simulink model "Get_Horizontal_Measures"  (R2014a)
settings: configuration reference "AR_Drone_ConfigSet" (kept outside this file)
undefined symbols (not defined in the file or in its folder): Accelerometer_360deg_calibration, Magnetometer_calibration, Navigation, Navigation_KF_Lib
libraries: simulink x7, AR_Drone_2_Library x1, vrlib x1
settings Model: SimulationMode=external  ExtModeTrigDuration=48000  Creator=nraman  LastModifiedBy=Raphaël

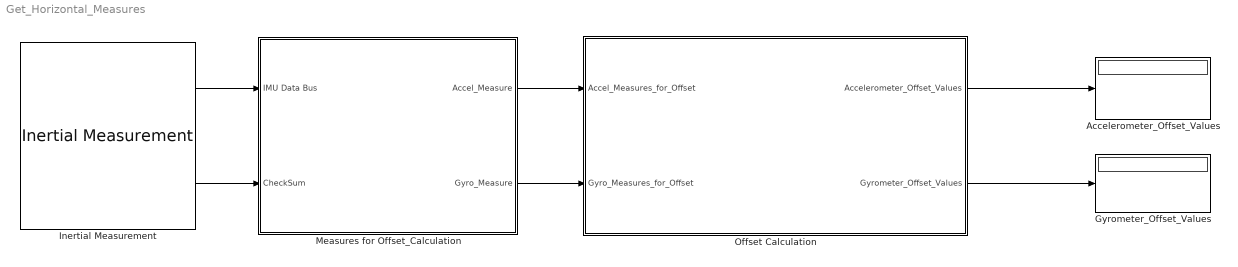
== system Get_Horizontal_Measures ==
  Accelerometer_Offset_Values : Display
      settings: Decimation=3
  Gyrometer_Offset_Values : Display
      settings: Decimation=3
  Inertial Measurement : AR_Drone_2_Library/Inertial Measurement  Ts=1/400
  Measures for Offset_Calculation : Subsystem  AncestorBlock=Navigation_KF_Lib/Navigation
      mask DialogControl DescTextVar Prompt: Kalman Filter Navigation Implementation
  Offset Calculation : Stateflow chart  RequirementInfo="{}  %GIDa_de274cbe_aff3_43d2_a93a_eae542baa43c"  TreatAsAtomicUnit=on
  wires:
  Inertial Measurement/1 -> Measures for Offset_Calculation/1(IMU Data Bus)
  Inertial Measurement/2 -> Measures for Offset_Calculation/2(CheckSum)
  Measures for Offset_Calculation/1(Accel_Measure) -> Offset Calculation/1(Accel_Measures_for_Offset)
  Measures for Offset_Calculation/2(Gyro_Measure) -> Offset Calculation/2(Gyro_Measures_for_Offset)
  Offset Calculation/2(Gyrometer_Offset_Values) -> Gyrometer_Offset_Values/1
  Offset Calculation/1(Accelerometer_Offset_Values) -> Accelerometer_Offset_Values/1

== system Get_Horizontal_Measures/Measures for Offset_Calculation ==
  IMU Data Bus : Inport  OutDataTypeStr=Bus: IMU_Packets
  CheckSum : Inport  Port=2
  Bus Creator1 : BusCreator  Inputs=5
  CheckSum Pre-Processing : Subsystem  TreatAsAtomicUnit=on
      settings: RTWSystemCode=Inline
  Data Conversion and Measurement Calculation : Subsystem
  Accel_Measure : Outport
  Gyro_Measure : Outport  Port=2
  wires:
  Bus Creator1/1 -> Data Conversion and Measurement Calculation/1(MeasurementDataBus)
  CheckSum Pre-Processing/5(GyroTemp_Measure) -> Bus Creator1/5  "GyroTemp_Measure"
  CheckSum Pre-Processing/4(Accelerometer_Measure) -> Bus Creator1/4  "Accelerometer_Measure"
  CheckSum Pre-Processing/3(BodyRates_Measure) -> Bus Creator1/3  "BodyRates_Measure"
  CheckSum Pre-Processing/2(Magnetometer_Measure) -> Bus Creator1/2  "Magnetometer_Measure"
  CheckSum Pre-Processing/1(UltraSoundHeight_Measure) -> Bus Creator1/1  "Ultrasound_Measure"
  CheckSum/1 -> CheckSum Pre-Processing/2(CheckSumFlag)
  IMU Data Bus/1 -> CheckSum Pre-Processing/1(IMU Packets)
  Data Conversion and Measurement Calculation/1(Accel_Measure) -> Accel_Measure/1
  Data Conversion and Measurement Calculation/2(Gyro_Measure) -> Gyro_Measure/1

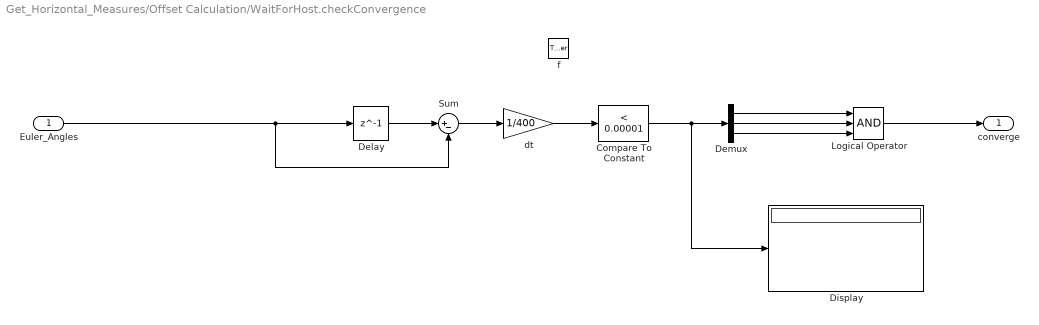
== system Get_Horizontal_Measures/Offset Calculation/WaitForHost.checkConvergence ==
  Euler_Angles : Inport  OutDataTypeStr=double  PortDimensions=3
  f : TriggerPort  TriggerType=function-call
      settings: CopyFcn=Stateflow.SLINSF.SimulinkMan.removeBlockPreDeleteFcn  PreDeleteFcn=Stateflow.SLINSF.SimulinkMan.unsafePredeleteFcn
  Compare To Constant : simulink/Logic and Bit Operations/Compare To Constant  relop=<  const=0.00001  OutDataTypeStr=boolean
  Delay : Delay  DelayLength=1  InitialCondition=inf
  Demux : Demux  Outputs=3
  Display : Display
  Logical Operator : Logic  Inputs=3  AllPortsSameDT=off  OutDataTypeStr=boolean
  Sum : Sum  Inputs=|+-
  dt : Gain  Gain=1/400
  converge : Outport
  wires:
  Euler_Angles/1 -> Sum/2, Delay/1
  Delay/1 -> Sum/1
  Sum/1 -> dt/1
  dt/1 -> Compare To Constant/1
  Compare To Constant/1 -> Display/1, Demux/1
  Logical Operator/1 -> converge/1
  Demux/1 -> Logical Operator/1
  Demux/2 -> Logical Operator/2
  Demux/3 -> Logical Operator/3

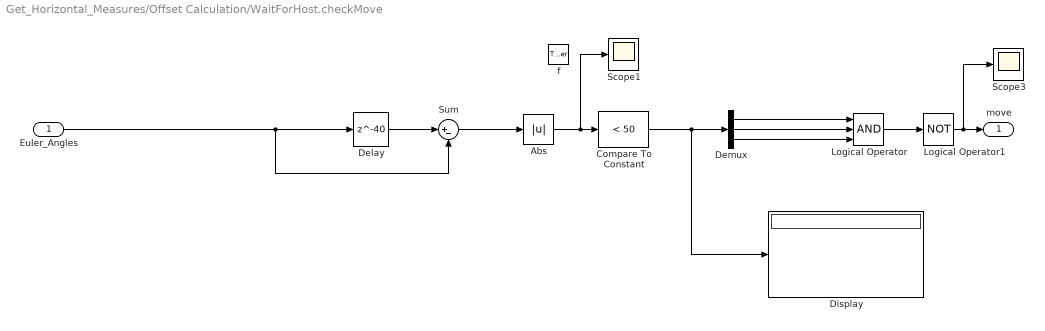
== system Get_Horizontal_Measures/Offset Calculation/WaitForHost.checkMove ==
  Euler_Angles : Inport  OutDataTypeStr=double  PortDimensions=3
  f : TriggerPort  TriggerType=function-call
      settings: CopyFcn=Stateflow.SLINSF.SimulinkMan.removeBlockPreDeleteFcn  PreDeleteFcn=Stateflow.SLINSF.SimulinkMan.unsafePredeleteFcn
  Abs : Abs
  Compare To Constant : simulink/Logic and Bit Operations/Compare To Constant  relop=<  const=50  OutDataTypeStr=boolean
  Delay : Delay  DelayLength=40  InitialCondition=inf
  Demux : Demux  Outputs=3
  Display : Display
  Logical Operator : Logic  Inputs=3  AllPortsSameDT=off  OutDataTypeStr=boolean
  Logical Operator1 : Logic  Operator=NOT  AllPortsSameDT=off  OutDataTypeStr=boolean
  Scope1 : Scope
      settings: SaveName=Difference
  Scope3 : Scope
      settings: SaveName=Move
  Sum : Sum  Inputs=|+-
  move : Outport
  wires:
  Euler_Angles/1 -> Sum/2, Delay/1
  Delay/1 -> Sum/1
  Sum/1 -> Abs/1
  Compare To Constant/1 -> Display/1, Demux/1
  Logical Operator/1 -> Logical Operator1/1
  Demux/1 -> Logical Operator/1
  Demux/2 -> Logical Operator/2
  Demux/3 -> Logical Operator/3
  Logical Operator1/1 -> Scope3/1, move/1
  Abs/1 -> Scope1/1, Compare To Constant/1

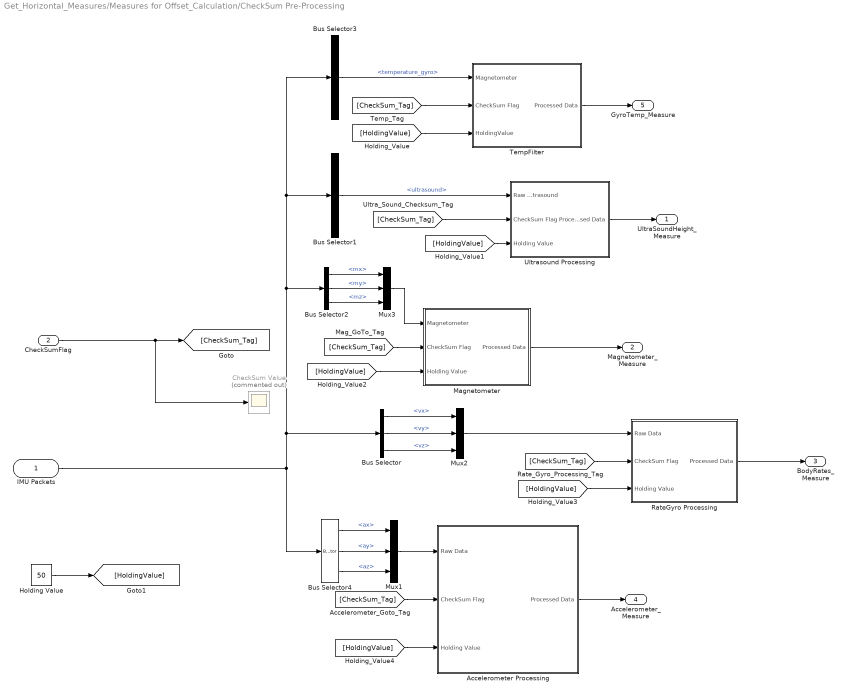
== system Get_Horizontal_Measures/Measures for Offset_Calculation/CheckSum Pre-Processing ==
  IMU Packets : Inport
  CheckSumFlag : Inport  Port=2
  Accelerometer Processing : Subsystem
  Bus Selector : BusSelector  OutputSignals=vx,vy,vz
  Bus Selector1 : BusSelector  OutputSignals=ultrasound
  Bus Selector2 : BusSelector  OutputSignals=mx,my,mz
  Bus Selector3 : BusSelector  OutputSignals=temperature_gyro
  Bus Selector4 : BusSelector  OutputSignals=ax,ay,az
  CheckSum Value : Scope  Commented=on
      settings: YMin=0  YMax=2500  SaveName=CheckSum
  Holding Value : Constant  Value=50
  Magnetometer : Subsystem
  Mux1 : Mux  Inputs=3
  Mux2 : Mux  Inputs=3
  Mux3 : Mux  Inputs=3
  RateGyro Processing : Subsystem
  TempFilter : Subsystem
  Ultrasound Processing : Subsystem
  UltraSoundHeight_Measure : Outport
  Magnetometer_Measure : Outport  Port=2
  BodyRates_Measure : Outport  Port=3
  Accelerometer_Measure : Outport  Port=4
  GyroTemp_Measure : Outport  Port=5
  wires:
  Mux3/1 -> Magnetometer/1(Magnetometer)
  Holding Value/1 -> [HoldingValue]
  [HoldingValue] -> Accelerometer Processing/3(Holding Value)
  [HoldingValue] -> RateGyro Processing/3(Holding Value)
  [HoldingValue] -> Magnetometer/3(Holding Value)
  [HoldingValue] -> Ultrasound Processing/3(Holding Value)
  [HoldingValue] -> TempFilter/3(HoldingValue)
  [CheckSum_Tag] -> TempFilter/2(CheckSum Flag)
  TempFilter/1(Processed Data) -> GyroTemp_Measure/1
  Bus Selector3/1 -> TempFilter/1(Magnetometer)  "<temperature_gyro>"
  Bus Selector/3 -> Mux2/3  "<vz>"
  Bus Selector/2 -> Mux2/2  "<vy>"
  Bus Selector/1 -> Mux2/1  "<vx>"
  Ultrasound Processing/1(Processed Data) -> UltraSoundHeight_Measure/1
  [CheckSum_Tag] -> Accelerometer Processing/2(CheckSum Flag)
  Magnetometer/1(Processed Data) -> Magnetometer_Measure/1
  [CheckSum_Tag] -> Magnetometer/2(CheckSum Flag)
  Bus Selector2/3 -> Mux3/3  "<mz>"
  Bus Selector2/2 -> Mux3/2  "<my>"
  Bus Selector2/1 -> Mux3/1  "<mx>"
  RateGyro Processing/1(Processed Data) -> BodyRates_Measure/1
  [CheckSum_Tag] -> RateGyro Processing/2(CheckSum Flag)
  Mux2/1 -> RateGyro Processing/1(Raw Data)
  Accelerometer Processing/1(Processed Data) -> Accelerometer_Measure/1
  [CheckSum_Tag] -> Ultrasound Processing/2(CheckSum Flag)
  Mux1/1 -> Accelerometer Processing/1(Raw Data)
  Bus Selector4/3 -> Mux1/3  "<az>"
  Bus Selector4/2 -> Mux1/2  "<ay>"
  Bus Selector4/1 -> Mux1/1  "<ax>"
  IMU Packets/1 -> Bus Selector4/1, Bus Selector2/1, Bus Selector1/1, Bus Selector3/1, Bus Selector/1
  CheckSumFlag/1 -> CheckSum Value/1, [CheckSum_Tag]
  Bus Selector1/1 -> Ultrasound Processing/1(Raw Ultrasound)  "<ultrasound>"

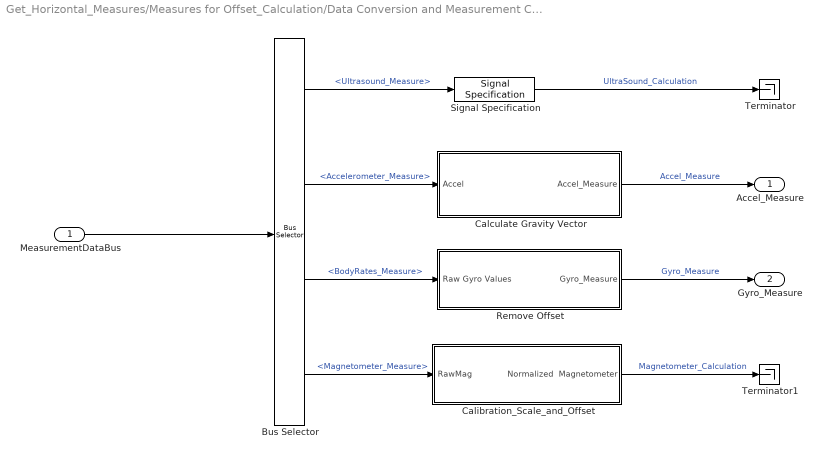
== system Get_Horizontal_Measures/Measures for Offset_Calculation/Data Conversion and Measurement Calculation ==
  MeasurementDataBus : Inport
  Bus Selector : BusSelector  OutputSignals=Ultrasound_Measure,Accelerometer_Measure,BodyRates_Measure,Magnetometer_Measure
  Calculate Gravity Vector : Subsystem
  Calibration_Scale_and_Offset : Subsystem
  Remove Offset : Subsystem
  Signal Specification : SignalSpecification
  Terminator : Terminator
  Terminator1 : Terminator
  Accel_Measure : Outport
  Gyro_Measure : Outport  Port=2
  wires:
  MeasurementDataBus/1 -> Bus Selector/1
  Bus Selector/4 -> Calibration_Scale_and_Offset/1(RawMag)  "<Magnetometer_Measure>"
  Bus Selector/3 -> Remove Offset/1(Raw Gyro Values)  "<BodyRates_Measure>"
  Bus Selector/1 -> Signal Specification/1  "<Ultrasound_Measure>"
  Calibration_Scale_and_Offset/1(Normalized  Magnetometer) -> Terminator1/1  "Magnetometer_Calculation"
  Remove Offset/1(Gyro_Measure) -> Gyro_Measure/1  "Gyro_Measure"
  Signal Specification/1 -> Terminator/1  "UltraSound_Calculation"
  Calculate Gravity Vector/1(Accel_Measure) -> Accel_Measure/1  "Accel_Measure"
  Bus Selector/2 -> Calculate Gravity Vector/1(Accel)  "<Accelerometer_Measure>"

== system Get_Horizontal_Measures/Measures for Offset_Calculation/CheckSum Pre-Processing/Accelerometer Processing ==
  Raw Data : Inport
  CheckSum Flag : Inport  Port=2
  Holding Value : Inport  Port=3
  Calculate Accel Data : Subsystem  Commented=through
  CheckSum Correction : Subsystem
  Processed Data : Outport
  wires:
  Holding Value/1 -> CheckSum Correction/3(Holding Value)
  Calculate Accel Data/1(Processed Accel Data) -> CheckSum Correction/1(CalculatedData)
  CheckSum Correction/1(Pre-Processed Height) -> Processed Data/1
  Raw Data/1 -> Calculate Accel Data/1(Raw Accel Data)
  CheckSum Flag/1 -> CheckSum Correction/2(CheckSumFlag)

== system Get_Horizontal_Measures/Measures for Offset_Calculation/CheckSum Pre-Processing/Magnetometer ==
  Magnetometer : Inport
  CheckSum Flag : Inport  Port=2
  Holding Value : Inport  Port=3
  CheckSum Correction : Subsystem
  Process Raw Mag Data : Subsystem  Commented=through
  Processed Data : Outport
  wires:
  Holding Value/1 -> CheckSum Correction/3(Holding Value)
  Process Raw Mag Data/1(ProcessedData) -> CheckSum Correction/1(CalculatedData)
  Magnetometer/1 -> Process Raw Mag Data/1(Magnetometer)
  CheckSum Correction/1(Pre-Processed Data) -> Processed Data/1
  CheckSum Flag/1 -> CheckSum Correction/2(CheckSumFlag)

== system Get_Horizontal_Measures/Measures for Offset_Calculation/CheckSum Pre-Processing/RateGyro Processing ==
  Raw Data : Inport
  CheckSum Flag : Inport  Port=2
  Holding Value : Inport  Port=3
  CheckSum Correction : Subsystem
  Process Data : Subsystem  Commented=through
  Processed Data : Outport
  wires:
  Holding Value/1 -> CheckSum Correction/3(Holding Value)
  Process Data/1(Processed Data) -> CheckSum Correction/1(CalculatedData)
  Raw Data/1 -> Process Data/1(Raw Data)
  CheckSum Correction/1(Pre-Processed Height) -> Processed Data/1
  CheckSum Flag/1 -> CheckSum Correction/2(CheckSumFlag)

== system Get_Horizontal_Measures/Measures for Offset_Calculation/CheckSum Pre-Processing/TempFilter ==
  Magnetometer : Inport
  CheckSum Flag : Inport  Port=2
  HoldingValue : Inport  Port=3
  CheckSum Correction : Subsystem
  Process Raw Mag Data : Subsystem  Commented=through
  Processed Data : Outport
  wires:
  HoldingValue/1 -> CheckSum Correction/3(Holding Value)
  Process Raw Mag Data/1(ProcessedData) -> CheckSum Correction/1(CalculatedData)
  Magnetometer/1 -> Process Raw Mag Data/1(Magnetometer)
  CheckSum Correction/1(Pre-Processed Data) -> Processed Data/1
  CheckSum Flag/1 -> CheckSum Correction/2(CheckSumFlag)

== system Get_Horizontal_Measures/Measures for Offset_Calculation/CheckSum Pre-Processing/Ultrasound Processing ==
  note: '192.168.1.1' 1 17725
  Raw Ultrasound : Inport
  CheckSum Flag : Inport  Port=2
  Holding Value : Inport  Port=3
  CheckSum Correction : Subsystem
  Data Type Conversion1 : DataTypeConversion
  Delay1 : Delay  DelayLength=1  InitialCondition=0
  Height Calculation : MATLAB Function  TreatAsAtomicUnit=on
  Saturation1 : Saturate  UpperLimit=100e3  LowerLimit=0
  Processed Data : Outport
  wires:
  Holding Value/1 -> CheckSum Correction/3(Holding Value)
  Saturation1/1 -> Processed Data/1
  CheckSum Correction/1(Pre-Processed Height) -> Saturation1/1
  CheckSum Flag/1 -> CheckSum Correction/2(CheckSumFlag)
  Height Calculation/1(y) -> CheckSum Correction/1(CalculatedData)
  Raw Ultrasound/1 -> Data Type Conversion1/1
  Height Calculation/2(prev_good_height) -> Delay1/1
  Data Type Conversion1/1 -> Height Calculation/1(u)
  Delay1/1 -> Height Calculation/2(z_1)

== system Get_Horizontal_Measures/Measures for Offset_Calculation/Data Conversion and Measurement Calculation/Calculate Gravity Vector ==
  Accel : Inport
  Accelerometer Neutral Gain and Offset : Subsystem
  Calibration_GainOffset : Subsystem
  Compare Calibration : Scope  NumInputPorts=2
      settings: TimeRange=6.848856838354834  YMin=-1.05~-1.05  YMax=0.05~0.1  SaveName=AccelProcessed_Record1
  Compare Offset : Scope  NumInputPorts=2
      settings: TimeRange=6.848856838354834  YMin=-0.05~-1  YMax=1.05~0.05  SaveName=AccelProcessed_Record
  InitialCondition_Offset : Subsystem
  Accel_Measure : Outport
  wires:
  Accelerometer Neutral Gain and Offset/1(Processed Accel Data) -> Compare Calibration/2, Calibration_GainOffset/1(Pre)
  Calibration_GainOffset/1(Post) -> Compare Offset/2, Compare Calibration/1, InitialCondition_Offset/1(Pre)
  Accel/1 -> Accelerometer Neutral Gain and Offset/1(Raw Accel Data)
  InitialCondition_Offset/1(Post) -> Accel_Measure/1, Compare Offset/1

== system Get_Horizontal_Measures/Measures for Offset_Calculation/Data Conversion and Measurement Calculation/Calibration_Scale_and_Offset ==
  RawMag : Inport
  Normalize Vector : vrlib/Utilities/Normalize Vector  maxzero=0
  Process Raw Mag Data : Subsystem  Variant=on  OverrideUsingVariant=TempVariantA
  Normalized  Magnetometer : Outport
  wires:
  Process Raw Mag Data/1(MagVector) -> Normalize Vector/1
  RawMag/1 -> Process Raw Mag Data/1(Magnetometer)
  Normalize Vector/1 -> Normalized  Magnetometer/1

== system Get_Horizontal_Measures/Measures for Offset_Calculation/Data Conversion and Measurement Calculation/Remove Offset ==
  Raw Gyro Values : Inport
  Gyro_Measure : Outport
  tag scope: Gyro_data_for_offset=global
  wires:
  Raw Gyro Values/1 -> Gyro_Measure/1, [Gyro_data_for_offset]

== system Get_Horizontal_Measures/Measures for Offset_Calculation/CheckSum Pre-Processing/Accelerometer Processing/Calculate Accel Data ==
  Raw Accel Data : Inport
  Bias : Constant  Value=[0 4096 4096]
  Gain : Gain  Gain=[0.001953125, 0.001953125, 0.001953125]
  Neutral Bias : Constant  Value=[2048 2048 2048]
  Sum : Sum  Inputs=|-+
  Sum1 : Sum  Inputs=|+-
  Processed Accel Data : Outport
  wires:
  Bias/1 -> Sum/2
  Neutral Bias/1 -> Sum1/2
  Sum/1 -> Sum1/1
  Gain/1 -> Processed Accel Data/1
  Sum1/1 -> Gain/1
  Raw Accel Data/1 -> Sum/1

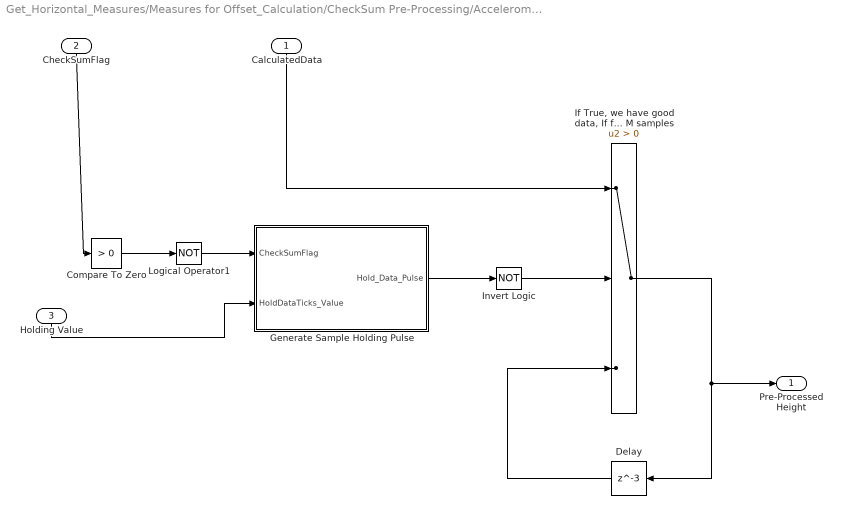
== system Get_Horizontal_Measures/Measures for Offset_Calculation/CheckSum Pre-Processing/Accelerometer Processing/CheckSum Correction ==
  CalculatedData : Inport
  CheckSumFlag : Inport  Port=2
  Holding Value : Inport  Port=3
  Compare To Zero : simulink/Logic and Bit Operations/Compare To Zero  relop=>  OutDataTypeStr=boolean
  Delay : Delay  DelayLength=3  InitialCondition=0
  Generate Sample Holding Pulse : Subsystem
  "If True, we have good data, If false, we have bad data, With bad data, use previous good data from N samples ago and hold it on that value for M samples" : Switch  Criteria=u2 > Threshold
  Invert Logic : Logic  Operator=NOT  AllPortsSameDT=off  OutDataTypeStr=boolean
  Logical Operator1 : Logic  Operator=NOT  AllPortsSameDT=off  OutDataTypeStr=boolean
  Pre-Processed Height : Outport
  wires:
  Holding Value/1 -> Generate Sample Holding Pulse/2(HoldDataTicks_Value)
  Invert Logic/1 -> "If True, we have good data, If false, we have bad data, With bad data, use previous good data from N samples ago and hold it on that value for M samples"/2
  Logical Operator1/1 -> Generate Sample Holding Pulse/1(CheckSumFlag)
  Generate Sample Holding Pulse/1(Hold_Data_Pulse) -> Invert Logic/1
  Compare To Zero/1 -> Logical Operator1/1
  Delay/1 -> "If True, we have good data, If false, we have bad data, With bad data, use previous good data from N samples ago and hold it on that value for M samples"/3
  "If True, we have good data, If false, we have bad data, With bad data, use previous good data from N samples ago and hold it on that value for M samples"/1 -> Delay/1, Pre-Processed Height/1
  CalculatedData/1 -> "If True, we have good data, If false, we have bad data, With bad data, use previous good data from N samples ago and hold it on that value for M samples"/1
  CheckSumFlag/1 -> Compare To Zero/1

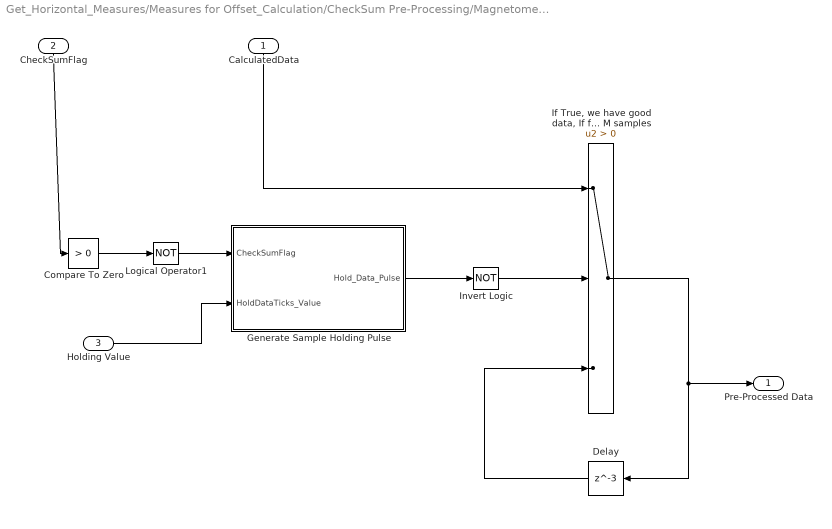
== system Get_Horizontal_Measures/Measures for Offset_Calculation/CheckSum Pre-Processing/Magnetometer/CheckSum Correction ==
  CalculatedData : Inport
  CheckSumFlag : Inport  Port=2
  Holding Value : Inport  Port=3
  Compare To Zero : simulink/Logic and Bit Operations/Compare To Zero  relop=>  OutDataTypeStr=boolean
  Delay : Delay  DelayLength=3  InitialCondition=0
  Generate Sample Holding Pulse : Subsystem
  "If True, we have good data, If false, we have bad data, With bad data, use previous good data from N samples ago and hold it on that value for M samples" : Switch  Criteria=u2 > Threshold
  Invert Logic : Logic  Operator=NOT  AllPortsSameDT=off  OutDataTypeStr=boolean
  Logical Operator1 : Logic  Operator=NOT  AllPortsSameDT=off  OutDataTypeStr=boolean
  Pre-Processed Data : Outport
  wires:
  Holding Value/1 -> Generate Sample Holding Pulse/2(HoldDataTicks_Value)
  Invert Logic/1 -> "If True, we have good data, If false, we have bad data, With bad data, use previous good data from N samples ago and hold it on that value for M samples"/2
  Logical Operator1/1 -> Generate Sample Holding Pulse/1(CheckSumFlag)
  Generate Sample Holding Pulse/1(Hold_Data_Pulse) -> Invert Logic/1
  Compare To Zero/1 -> Logical Operator1/1
  Delay/1 -> "If True, we have good data, If false, we have bad data, With bad data, use previous good data from N samples ago and hold it on that value for M samples"/3
  "If True, we have good data, If false, we have bad data, With bad data, use previous good data from N samples ago and hold it on that value for M samples"/1 -> Delay/1, Pre-Processed Data/1
  CalculatedData/1 -> "If True, we have good data, If false, we have bad data, With bad data, use previous good data from N samples ago and hold it on that value for M samples"/1
  CheckSumFlag/1 -> Compare To Zero/1

== system Get_Horizontal_Measures/Measures for Offset_Calculation/CheckSum Pre-Processing/Magnetometer/Process Raw Mag Data ==
  note: magnetometer[ 0 ] = - ( float ) navdata.mx ;
      | magnetometer[ 1 ] = ( float ) navdata.my ;
      | magnetometer[ 2 ] = - ( float ) navdata.mz ;
      | const float Sensitivity[ 3 ] = { 0.0071492608 , 0.0070882491 , 0.0074057781 } ;
      | const float Neutral[ 3 ] = { 118.0 , - 65.0 , 110.0 } ;
  Magnetometer : Inport
  Bias : Constant  Value=[ 118.0, -65.0, 110.0 ]
  Sum : Sum  Inputs=|+-
  postGain : Gain  Gain=[0.0071492608, 0.0070882491, 0.0074057781]
  preGain : Gain  Gain=[-1 1 -1]
  ProcessedData : Outport
  wires:
  Bias/1 -> Sum/2
  preGain/1 -> Sum/1
  Sum/1 -> postGain/1
  Magnetometer/1 -> preGain/1
  postGain/1 -> ProcessedData/1

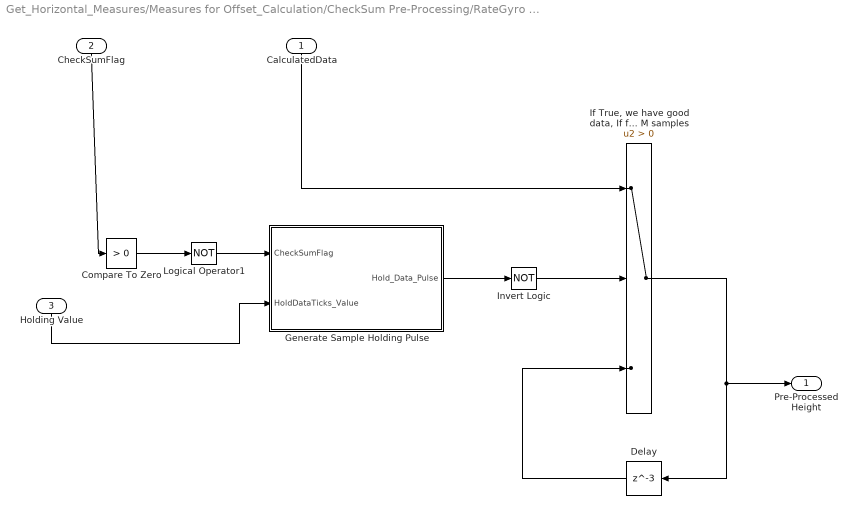
== system Get_Horizontal_Measures/Measures for Offset_Calculation/CheckSum Pre-Processing/RateGyro Processing/CheckSum Correction ==
  CalculatedData : Inport
  CheckSumFlag : Inport  Port=2
  Holding Value : Inport  Port=3
  Compare To Zero : simulink/Logic and Bit Operations/Compare To Zero  relop=>  OutDataTypeStr=boolean
  Delay : Delay  DelayLength=3  InitialCondition=0
  Generate Sample Holding Pulse : Subsystem
  "If True, we have good data, If false, we have bad data, With bad data, use previous good data from N samples ago and hold it on that value for M samples" : Switch  Criteria=u2 > Threshold
  Invert Logic : Logic  Operator=NOT  AllPortsSameDT=off  OutDataTypeStr=boolean
  Logical Operator1 : Logic  Operator=NOT  AllPortsSameDT=off  OutDataTypeStr=boolean
  Pre-Processed Height : Outport
  wires:
  Holding Value/1 -> Generate Sample Holding Pulse/2(HoldDataTicks_Value)
  Invert Logic/1 -> "If True, we have good data, If false, we have bad data, With bad data, use previous good data from N samples ago and hold it on that value for M samples"/2
  Logical Operator1/1 -> Generate Sample Holding Pulse/1(CheckSumFlag)
  Generate Sample Holding Pulse/1(Hold_Data_Pulse) -> Invert Logic/1
  Compare To Zero/1 -> Logical Operator1/1
  Delay/1 -> "If True, we have good data, If false, we have bad data, With bad data, use previous good data from N samples ago and hold it on that value for M samples"/3
  "If True, we have good data, If false, we have bad data, With bad data, use previous good data from N samples ago and hold it on that value for M samples"/1 -> Delay/1, Pre-Processed Height/1
  CalculatedData/1 -> "If True, we have good data, If false, we have bad data, With bad data, use previous good data from N samples ago and hold it on that value for M samples"/1
  CheckSumFlag/1 -> Compare To Zero/1

== system Get_Horizontal_Measures/Measures for Offset_Calculation/CheckSum Pre-Processing/RateGyro Processing/Process Data ==
  note: const float Sensitivity[ 3 ] = { 0.0609 , 0.0609 , 0.0609 } ;
      | const float Neutral[ 3 ] = { 0.0 , 0.0 , 0.0 } ;
      | const int16_t Offset[ 3 ] = { - 73 , 14 , - 13 } ;
      | const int16_t Noises[ 3 ] = { 35 , 35 , 15 } ;
      |
      | int16_t vRaws[ 3 ] = {
      | Navdata :: IMU :: Gyroscope :: getRawX (),
      | Navdata :: IMU :: Gyroscope :: getRawY (),
      | Navdata :: IMU :: Gyroscope :: getRawZ ()
      | } ;
      |
      | gyroscope[i] = vRaws[i] * Gyroscope :: Sensitivity[i] * M_PI / 180.0 ;
  Raw Data : Inport
  Constant : Constant  Value=[0.0, 0.0, 0.0]
  Gain : Gain  Gain=[0.0609, 0.0609, 0.0609]
  Sum : Sum  Inputs=|++
  Processed Data : Outport
  wires:
  Raw Data/1 -> Sum/1
  Constant/1 -> Sum/2
  Gain/1 -> Processed Data/1
  Sum/1 -> Gain/1

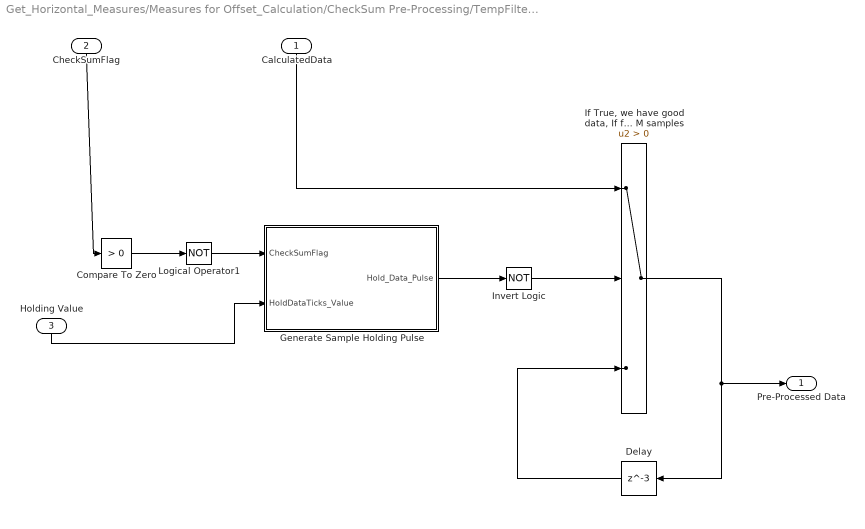
== system Get_Horizontal_Measures/Measures for Offset_Calculation/CheckSum Pre-Processing/TempFilter/CheckSum Correction ==
  CalculatedData : Inport
  CheckSumFlag : Inport  Port=2
  Holding Value : Inport  Port=3
  Compare To Zero : simulink/Logic and Bit Operations/Compare To Zero  relop=>  OutDataTypeStr=boolean
  Delay : Delay  DelayLength=3  InitialCondition=0
  Generate Sample Holding Pulse : Subsystem
  "If True, we have good data, If false, we have bad data, With bad data, use previous good data from N samples ago and hold it on that value for M samples" : Switch  Criteria=u2 > Threshold
  Invert Logic : Logic  Operator=NOT  AllPortsSameDT=off  OutDataTypeStr=boolean
  Logical Operator1 : Logic  Operator=NOT  AllPortsSameDT=off  OutDataTypeStr=boolean
  Pre-Processed Data : Outport
  wires:
  Holding Value/1 -> Generate Sample Holding Pulse/2(HoldDataTicks_Value)
  Invert Logic/1 -> "If True, we have good data, If false, we have bad data, With bad data, use previous good data from N samples ago and hold it on that value for M samples"/2
  Logical Operator1/1 -> Generate Sample Holding Pulse/1(CheckSumFlag)
  Generate Sample Holding Pulse/1(Hold_Data_Pulse) -> Invert Logic/1
  Compare To Zero/1 -> Logical Operator1/1
  Delay/1 -> "If True, we have good data, If false, we have bad data, With bad data, use previous good data from N samples ago and hold it on that value for M samples"/3
  "If True, we have good data, If false, we have bad data, With bad data, use previous good data from N samples ago and hold it on that value for M samples"/1 -> Delay/1, Pre-Processed Data/1
  CalculatedData/1 -> "If True, we have good data, If false, we have bad data, With bad data, use previous good data from N samples ago and hold it on that value for M samples"/1
  CheckSumFlag/1 -> Compare To Zero/1

== system Get_Horizontal_Measures/Measures for Offset_Calculation/CheckSum Pre-Processing/TempFilter/Process Raw Mag Data ==
  note: magnetometer[ 0 ] = - ( float ) navdata.mx ;
      | magnetometer[ 1 ] = ( float ) navdata.my ;
      | magnetometer[ 2 ] = - ( float ) navdata.mz ;
      | const float Sensitivity[ 3 ] = { 0.0071492608 , 0.0070882491 , 0.0074057781 } ;
      | const float Neutral[ 3 ] = { 118.0 , - 65.0 , 110.0 } ;
  Magnetometer : Inport
  Bias : Constant  Value=[ 118.0, -65.0, 110.0 ]
  Sum : Sum  Inputs=|+-
  postGain : Gain  Gain=[0.0071492608, 0.0070882491, 0.0074057781]
  preGain : Gain  Gain=[-1 1 -1]
  ProcessedData : Outport
  wires:
  Bias/1 -> Sum/2
  preGain/1 -> Sum/1
  Sum/1 -> postGain/1
  Magnetometer/1 -> preGain/1
  postGain/1 -> ProcessedData/1

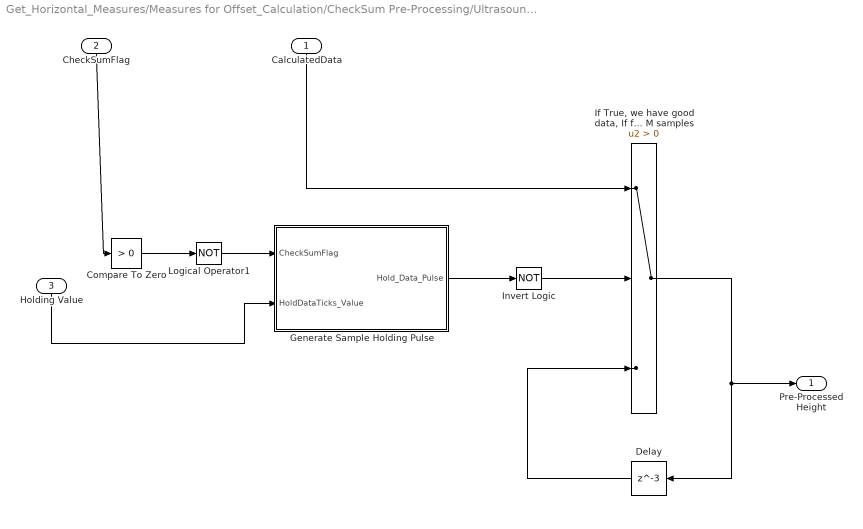
== system Get_Horizontal_Measures/Measures for Offset_Calculation/CheckSum Pre-Processing/Ultrasound Processing/CheckSum Correction ==
  CalculatedData : Inport
  CheckSumFlag : Inport  Port=2
  Holding Value : Inport  Port=3
  Compare To Zero : simulink/Logic and Bit Operations/Compare To Zero  relop=>  OutDataTypeStr=boolean
  Delay : Delay  DelayLength=3  InitialCondition=0
  Generate Sample Holding Pulse : Subsystem
  "If True, we have good data, If false, we have bad data, With bad data, use previous good data from N samples ago and hold it on that value for M samples" : Switch  Criteria=u2 > Threshold
  Invert Logic : Logic  Operator=NOT  AllPortsSameDT=off  OutDataTypeStr=boolean
  Logical Operator1 : Logic  Operator=NOT  AllPortsSameDT=off  OutDataTypeStr=boolean
  Pre-Processed Height : Outport
  wires:
  Holding Value/1 -> Generate Sample Holding Pulse/2(HoldDataTicks_Value)
  Invert Logic/1 -> "If True, we have good data, If false, we have bad data, With bad data, use previous good data from N samples ago and hold it on that value for M samples"/2
  Logical Operator1/1 -> Generate Sample Holding Pulse/1(CheckSumFlag)
  Generate Sample Holding Pulse/1(Hold_Data_Pulse) -> Invert Logic/1
  Compare To Zero/1 -> Logical Operator1/1
  Delay/1 -> "If True, we have good data, If false, we have bad data, With bad data, use previous good data from N samples ago and hold it on that value for M samples"/3
  "If True, we have good data, If false, we have bad data, With bad data, use previous good data from N samples ago and hold it on that value for M samples"/1 -> Delay/1, Pre-Processed Height/1
  CalculatedData/1 -> "If True, we have good data, If false, we have bad data, With bad data, use previous good data from N samples ago and hold it on that value for M samples"/1
  CheckSumFlag/1 -> Compare To Zero/1

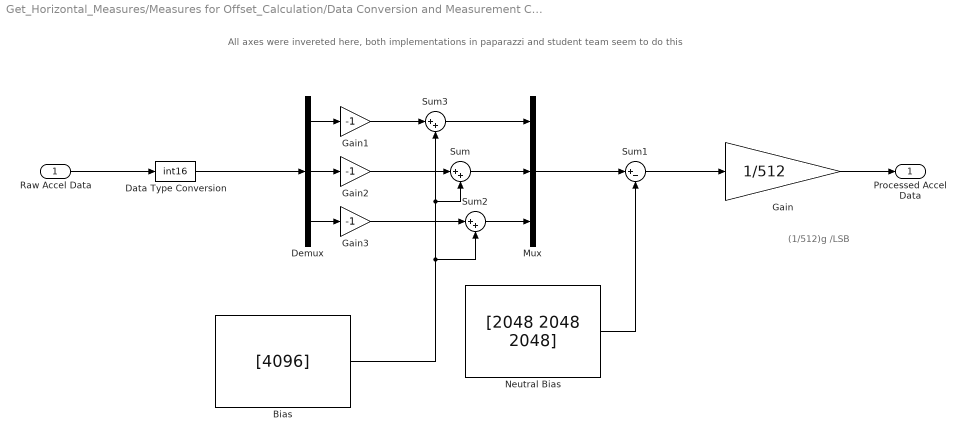
== system Get_Horizontal_Measures/Measures for Offset_Calculation/Data Conversion and Measurement Calculation/Calculate Gravity Vector/Accelerometer Neutral Gain and Offset ==
  note: (1/512)g /LSB
  note: All axes were invereted here, both implementations in paparazzi and student team seem to do this
  Raw Accel Data : Inport
  Bias : Constant  Value=[4096]
  Data Type Conversion : DataTypeConversion  OutDataTypeStr=int16
  Demux : Demux  Outputs=3
  Gain : Gain  Gain=1/512
  Gain1 : Gain  Gain=-1  OutDataTypeStr=double
  Gain2 : Gain  Gain=-1  OutDataTypeStr=double
  Gain3 : Gain  Gain=-1  OutDataTypeStr=double
  Mux : Mux  Inputs=3
  Neutral Bias : Constant  Value=[2048 2048 2048]
  Sum : Sum  Inputs=|++
  Sum1 : Sum  Inputs=|+-
  Sum2 : Sum  Inputs=|++
  Sum3 : Sum  Inputs=|++
  Processed Accel Data : Outport
  wires:
  Gain1/1 -> Sum3/1
  Data Type Conversion/1 -> Demux/1
  Bias/1 -> Sum3/2, Sum/2, Sum2/2
  Sum2/1 -> Mux/3
  Gain3/1 -> Sum2/1
  Demux/3 -> Gain3/1
  Sum/1 -> Mux/2
  Gain2/1 -> Sum/1
  Demux/2 -> Gain2/1
  Sum3/1 -> Mux/1
  Demux/1 -> Gain1/1
  Raw Accel Data/1 -> Data Type Conversion/1
  Neutral Bias/1 -> Sum1/2
  Mux/1 -> Sum1/1
  Gain/1 -> Processed Accel Data/1
  Sum1/1 -> Gain/1

== system Get_Horizontal_Measures/Measures for Offset_Calculation/Data Conversion and Measurement Calculation/Calculate Gravity Vector/Calibration_GainOffset ==
  Pre : Inport
  Accel_Calib_Gain : Constant  Value=Accelerometer_360deg_calibration.Gains
      settings: AttributesFormatString=%<Value>
  Accel_Calib_Offset : Constant  Value=Accelerometer_360deg_calibration.Offsets
      settings: AttributesFormatString=%<Value>
  Gain : Gain  Gain=-1  OutDataTypeStr=Inherit: Same as input
  Multiply : Product  Inputs=*/
  Sum : Sum  Inputs=|+-
  Post : Outport
  wires:
  Gain/1 -> Multiply/2
  Accel_Calib_Gain/1 -> Gain/1
  Pre/1 -> Sum/1
  Sum/1 -> Multiply/1
  Accel_Calib_Offset/1 -> Sum/2
  Multiply/1 -> Post/1

== system Get_Horizontal_Measures/Measures for Offset_Calculation/Data Conversion and Measurement Calculation/Calculate Gravity Vector/InitialCondition_Offset ==
  Pre : Inport
  Post : Outport
  tag scope: Accel_data_for_offset=global
  wires:
  Pre/1 -> Post/1, [Accel_data_for_offset]

== system Get_Horizontal_Measures/Measures for Offset_Calculation/Data Conversion and Measurement Calculation/Calibration_Scale_and_Offset/Process Raw Mag Data ==
  Magnetometer : Inport
  Process Raw Mag Data (Home_330453) : Subsystem  VariantControl=TempVariantA
  Process Raw Mag Data (Work_255725) : Subsystem  VariantControl=TempVariantB
  MagVector : Outport

== system Get_Horizontal_Measures/Measures for Offset_Calculation/CheckSum Pre-Processing/Accelerometer Processing/CheckSum Correction/Generate Sample Holding Pulse ==
  CheckSumFlag : Inport
  HoldDataTicks_Value : Inport  Port=2
  Chart : Stateflow chart  TreatAsAtomicUnit=on
  Constant2 : Constant
  Logical Operator1 : Logic  AllPortsSameDT=off  OutDataTypeStr=boolean
  Transition Logic Detection : Subsystem
  Hold_Data_Pulse : Outport
  wires:
  HoldDataTicks_Value/1 -> Chart/2(HoldDataTicks)
  CheckSumFlag/1 -> Transition Logic Detection/1(Input)
  Transition Logic Detection/1(Transition Detect) -> Chart/1(if_transition)
  Chart/1(output) -> Logical Operator1/2
  Logical Operator1/1 -> Hold_Data_Pulse/1
  Constant2/1 -> Logical Operator1/1

== system Get_Horizontal_Measures/Measures for Offset_Calculation/CheckSum Pre-Processing/Magnetometer/CheckSum Correction/Generate Sample Holding Pulse ==
  CheckSumFlag : Inport
  HoldDataTicks_Value : Inport  Port=2
  Chart : Stateflow chart  TreatAsAtomicUnit=on
  Constant2 : Constant
  Logical Operator1 : Logic  AllPortsSameDT=off  OutDataTypeStr=boolean
  Transition Logic Detection : Subsystem
  Hold_Data_Pulse : Outport
  wires:
  HoldDataTicks_Value/1 -> Chart/2(HoldDataTicks)
  CheckSumFlag/1 -> Transition Logic Detection/1(Input)
  Transition Logic Detection/1(Transition Detect) -> Chart/1(if_transition)
  Chart/1(output) -> Logical Operator1/2
  Logical Operator1/1 -> Hold_Data_Pulse/1
  Constant2/1 -> Logical Operator1/1

== system Get_Horizontal_Measures/Measures for Offset_Calculation/CheckSum Pre-Processing/RateGyro Processing/CheckSum Correction/Generate Sample Holding Pulse ==
  CheckSumFlag : Inport
  HoldDataTicks_Value : Inport  Port=2
  Chart : Stateflow chart  TreatAsAtomicUnit=on
  Constant2 : Constant
  Logical Operator1 : Logic  AllPortsSameDT=off  OutDataTypeStr=boolean
  Transition Logic Detection : Subsystem
  Hold_Data_Pulse : Outport
  wires:
  HoldDataTicks_Value/1 -> Chart/2(HoldDataTicks)
  CheckSumFlag/1 -> Transition Logic Detection/1(Input)
  Transition Logic Detection/1(Transition Detect) -> Chart/1(if_transition)
  Chart/1(output) -> Logical Operator1/2
  Logical Operator1/1 -> Hold_Data_Pulse/1
  Constant2/1 -> Logical Operator1/1

== system Get_Horizontal_Measures/Measures for Offset_Calculation/CheckSum Pre-Processing/TempFilter/CheckSum Correction/Generate Sample Holding Pulse ==
  CheckSumFlag : Inport
  HoldDataTicks_Value : Inport  Port=2
  Chart : Stateflow chart  TreatAsAtomicUnit=on
  Constant2 : Constant
  Logical Operator1 : Logic  AllPortsSameDT=off  OutDataTypeStr=boolean
  Transition Logic Detection : Subsystem
  Hold_Data_Pulse : Outport
  wires:
  HoldDataTicks_Value/1 -> Chart/2(HoldDataTicks)
  CheckSumFlag/1 -> Transition Logic Detection/1(Input)
  Transition Logic Detection/1(Transition Detect) -> Chart/1(if_transition)
  Chart/1(output) -> Logical Operator1/2
  Logical Operator1/1 -> Hold_Data_Pulse/1
  Constant2/1 -> Logical Operator1/1

== system Get_Horizontal_Measures/Measures for Offset_Calculation/CheckSum Pre-Processing/Ultrasound Processing/CheckSum Correction/Generate Sample Holding Pulse ==
  CheckSumFlag : Inport
  HoldDataTicks_Value : Inport  Port=2
  Chart : Stateflow chart  TreatAsAtomicUnit=on
  Constant2 : Constant
  Logical Operator1 : Logic  AllPortsSameDT=off  OutDataTypeStr=boolean
  Transition Logic Detection : Subsystem
  Hold_Data_Pulse : Outport
  wires:
  HoldDataTicks_Value/1 -> Chart/2(HoldDataTicks)
  CheckSumFlag/1 -> Transition Logic Detection/1(Input)
  Transition Logic Detection/1(Transition Detect) -> Chart/1(if_transition)
  Chart/1(output) -> Logical Operator1/2
  Logical Operator1/1 -> Hold_Data_Pulse/1
  Constant2/1 -> Logical Operator1/1

== system Get_Horizontal_Measures/Measures for Offset_Calculation/Data Conversion and Measurement Calculation/Calibration_Scale_and_Offset/Process Raw Mag Data/Process Raw Mag Data (Home_330453) ==
  note: magnetometer[ 0 ] = - ( float ) navdata.mx ;
      | magnetometer[ 1 ] = ( float ) navdata.my ;
      | magnetometer[ 2 ] = - ( float ) navdata.mz ;
      | const float Sensitivity[ 3 ] = { 0.0071492608 , 0.0070882491 , 0.0074057781 } ;
      | const float Neutral[ 3 ] = { 118.0 , - 65.0 , 110.0 } ;
  Magnetometer : Inport
  Bias : Constant  Commented=on  Value=[-23 4.3 1.44]
  Constant : Constant  Value=Magnetometer_calibration.Offsets
      settings: AttributesFormatString=%<Value>
  Constant1 : Constant  Value=Magnetometer_calibration.Gains
      settings: AttributesFormatString=%<Value>
  Divide : Product  Inputs=/*
  Sum : Sum  Inputs=|+-
  postGain : Gain  Commented=on  Gain=1./[187 163 139]
  MagVector : Outport
  wires:
  Constant1/1 -> Divide/1
  Sum/1 -> Divide/2
  Magnetometer/1 -> Sum/1
  Constant/1 -> Sum/2
  Divide/1 -> MagVector/1

== system Get_Horizontal_Measures/Measures for Offset_Calculation/Data Conversion and Measurement Calculation/Calibration_Scale_and_Offset/Process Raw Mag Data/Process Raw Mag Data (Work_255725) ==
  note: 158 145 136
  note: magnetometer[ 0 ] = - ( float ) navdata.mx ;
      | magnetometer[ 1 ] = ( float ) navdata.my ;
      | magnetometer[ 2 ] = - ( float ) navdata.mz ;
      | const float Sensitivity[ 3 ] = { 0.0071492608 , 0.0070882491 , 0.0074057781 } ;
      | const float Neutral[ 3 ] = { 118.0 , - 65.0 , 110.0 } ;
  Magnetometer : Inport
  Bias : Constant  Value=[2.93 18.9 77.5]
  Low Pass Filter1 : Subsystem  Commented=through
      mask Display: disp(['Elliptic Filter with 20 Hz corner', '\n', '44 dB stopband.'])
  Sum : Sum  Inputs=|+-
  postGain : Gain  Gain=1./[167 135 132]
  preGain : Gain  Commented=through  Gain=[1 1 1]
  MagVector : Outport
  wires:
  postGain/1 -> Low Pass Filter1/1(Input)
  Magnetometer/1 -> preGain/1
  Sum/1 -> postGain/1
  preGain/1 -> Sum/1
  Bias/1 -> Sum/2
  Low Pass Filter1/1(Output) -> MagVector/1

== system Get_Horizontal_Measures/Measures for Offset_Calculation/CheckSum Pre-Processing/Accelerometer Processing/CheckSum Correction/Generate Sample Holding Pulse/Transition Logic Detection ==
  Input : Inport
  Constant : Constant  Value=0
  Constant1 : Constant
  Logical Operator : Logic  AllPortsSameDT=off  OutDataTypeStr=boolean
  Relational Operator : RelationalOperator  Operator===  OutDataTypeStr=boolean
  Relational Operator1 : RelationalOperator  Operator===  OutDataTypeStr=boolean
  Unit Delay : UnitDelay  SampleTime=-1
  Transition Detect : Outport
  wires:
  Logical Operator/1 -> Transition Detect/1  "Transition_Detect"
  Constant1/1 -> Relational Operator1/1
  Constant/1 -> Relational Operator/2
  Relational Operator/1 -> Logical Operator/2
  Input/1 -> Unit Delay/1, Relational Operator1/2
  Unit Delay/1 -> Relational Operator/1
  Relational Operator1/1 -> Logical Operator/1

== system Get_Horizontal_Measures/Measures for Offset_Calculation/CheckSum Pre-Processing/Magnetometer/CheckSum Correction/Generate Sample Holding Pulse/Transition Logic Detection ==
  Input : Inport
  Constant : Constant  Value=0
  Constant1 : Constant
  Logical Operator : Logic  AllPortsSameDT=off  OutDataTypeStr=boolean
  Relational Operator : RelationalOperator  Operator===  OutDataTypeStr=boolean
  Relational Operator1 : RelationalOperator  Operator===  OutDataTypeStr=boolean
  Unit Delay : UnitDelay  SampleTime=-1
  Transition Detect : Outport
  wires:
  Logical Operator/1 -> Transition Detect/1  "Transition_Detect"
  Constant1/1 -> Relational Operator1/1
  Constant/1 -> Relational Operator/2
  Relational Operator/1 -> Logical Operator/2
  Input/1 -> Unit Delay/1, Relational Operator1/2
  Unit Delay/1 -> Relational Operator/1
  Relational Operator1/1 -> Logical Operator/1

== system Get_Horizontal_Measures/Measures for Offset_Calculation/CheckSum Pre-Processing/RateGyro Processing/CheckSum Correction/Generate Sample Holding Pulse/Transition Logic Detection ==
  Input : Inport
  Constant : Constant  Value=0
  Constant1 : Constant
  Logical Operator : Logic  AllPortsSameDT=off  OutDataTypeStr=boolean
  Relational Operator : RelationalOperator  Operator===  OutDataTypeStr=boolean
  Relational Operator1 : RelationalOperator  Operator===  OutDataTypeStr=boolean
  Unit Delay : UnitDelay  SampleTime=-1
  Transition Detect : Outport
  wires:
  Logical Operator/1 -> Transition Detect/1  "Transition_Detect"
  Constant1/1 -> Relational Operator1/1
  Constant/1 -> Relational Operator/2
  Relational Operator/1 -> Logical Operator/2
  Input/1 -> Unit Delay/1, Relational Operator1/2
  Unit Delay/1 -> Relational Operator/1
  Relational Operator1/1 -> Logical Operator/1

== system Get_Horizontal_Measures/Measures for Offset_Calculation/CheckSum Pre-Processing/TempFilter/CheckSum Correction/Generate Sample Holding Pulse/Transition Logic Detection ==
  Input : Inport
  Constant : Constant  Value=0
  Constant1 : Constant
  Logical Operator : Logic  AllPortsSameDT=off  OutDataTypeStr=boolean
  Relational Operator : RelationalOperator  Operator===  OutDataTypeStr=boolean
  Relational Operator1 : RelationalOperator  Operator===  OutDataTypeStr=boolean
  Unit Delay : UnitDelay  SampleTime=-1
  Transition Detect : Outport
  wires:
  Logical Operator/1 -> Transition Detect/1  "Transition_Detect"
  Constant1/1 -> Relational Operator1/1
  Constant/1 -> Relational Operator/2
  Relational Operator/1 -> Logical Operator/2
  Input/1 -> Unit Delay/1, Relational Operator1/2
  Unit Delay/1 -> Relational Operator/1
  Relational Operator1/1 -> Logical Operator/1

== system Get_Horizontal_Measures/Measures for Offset_Calculation/CheckSum Pre-Processing/Ultrasound Processing/CheckSum Correction/Generate Sample Holding Pulse/Transition Logic Detection ==
  Input : Inport
  Constant : Constant  Value=0
  Constant1 : Constant
  Logical Operator : Logic  AllPortsSameDT=off  OutDataTypeStr=boolean
  Relational Operator : RelationalOperator  Operator===  OutDataTypeStr=boolean
  Relational Operator1 : RelationalOperator  Operator===  OutDataTypeStr=boolean
  Unit Delay : UnitDelay  SampleTime=-1
  Transition Detect : Outport
  wires:
  Logical Operator/1 -> Transition Detect/1  "Transition_Detect"
  Constant1/1 -> Relational Operator1/1
  Constant/1 -> Relational Operator/2
  Relational Operator/1 -> Logical Operator/2
  Input/1 -> Unit Delay/1, Relational Operator1/2
  Unit Delay/1 -> Relational Operator/1
  Relational Operator1/1 -> Logical Operator/1

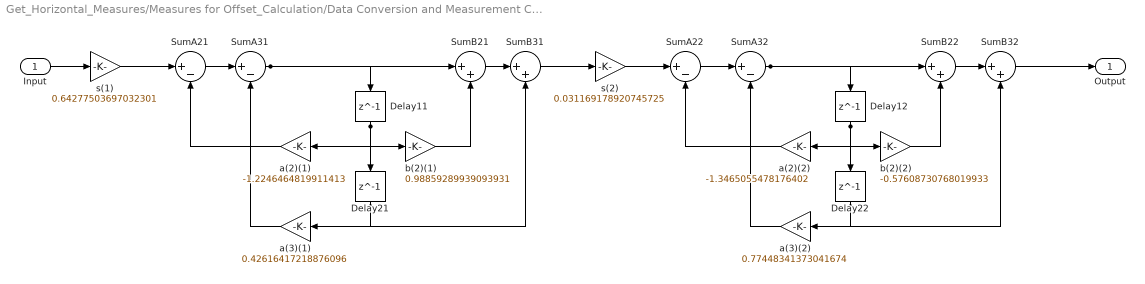
== system Get_Horizontal_Measures/Measures for Offset_Calculation/Data Conversion and Measurement Calculation/Calibration_Scale_and_Offset/Process Raw Mag Data/Process Raw Mag Data (Work_255725)/Low Pass Filter1 ==
  Input : Inport
  Delay{11..12,21..22} (4 alike) : Delay  DelayLength=1  InitialCondition=0
  SumA{21..22,31..32} (4 alike) : Sum  Inputs=|+-  RndMeth=Nearest  SaturateOnIntegerOverflow=on  OutDataTypeStr=Inherit: Same as first input
  SumB{21..22,31..32} (4 alike) : Sum  Inputs=|++  RndMeth=Nearest  SaturateOnIntegerOverflow=on  OutDataTypeStr=Inherit: Same as first input
  a(2)(1) : Gain  Gain=-1.2246464819911413  ParamDataTypeStr=double  RndMeth=Nearest  SaturateOnIntegerOverflow=on  OutDataTypeStr=Inherit: Same as input
  a(2)(2) : Gain  Gain=-1.3465055478176402  ParamDataTypeStr=double  RndMeth=Nearest  SaturateOnIntegerOverflow=on  OutDataTypeStr=Inherit: Same as input
  a(3)(1) : Gain  Gain=0.42616417218876096  ParamDataTypeStr=double  RndMeth=Nearest  SaturateOnIntegerOverflow=on  OutDataTypeStr=Inherit: Same as input
  a(3)(2) : Gain  Gain=0.77448341373041674  ParamDataTypeStr=double  RndMeth=Nearest  SaturateOnIntegerOverflow=on  OutDataTypeStr=Inherit: Same as input
  b(2)(1) : Gain  Gain=0.98859289939093931  ParamDataTypeStr=double  RndMeth=Nearest  SaturateOnIntegerOverflow=on  OutDataTypeStr=Inherit: Same as input
  b(2)(2) : Gain  Gain=-0.57608730768019933  ParamDataTypeStr=double  RndMeth=Nearest  SaturateOnIntegerOverflow=on  OutDataTypeStr=Inherit: Same as input
  s(1) : Gain  Gain=0.64277503697032301  ParamDataTypeStr=double  RndMeth=Nearest  SaturateOnIntegerOverflow=on  OutDataTypeStr=Inherit: Same as input
  s(2) : Gain  Gain=0.031169178920745725  ParamDataTypeStr=double  RndMeth=Nearest  SaturateOnIntegerOverflow=on  OutDataTypeStr=Inherit: Same as input
  Output : Outport
  wires:
  Delay22/1 -> SumB32/2, a(3)(2)/1
  a(3)(2)/1 -> SumA32/2
  b(2)(2)/1 -> SumB22/2
  Delay12/1 -> Delay22/1, b(2)(2)/1, a(2)(2)/1
  a(2)(2)/1 -> SumA22/2
  SumB32/1 -> Output/1
  SumB22/1 -> SumB32/1
  SumA32/1 -> Delay12/1, SumB22/1
  SumA22/1 -> SumA32/1
  s(2)/1 -> SumA22/1
  Delay21/1 -> SumB31/2, a(3)(1)/1
  a(3)(1)/1 -> SumA31/2
  b(2)(1)/1 -> SumB21/2
  Delay11/1 -> Delay21/1, b(2)(1)/1, a(2)(1)/1
  a(2)(1)/1 -> SumA21/2
  SumB31/1 -> s(2)/1
  SumB21/1 -> SumB31/1
  SumA31/1 -> Delay11/1, SumB21/1
  SumA21/1 -> SumA31/1
  s(1)/1 -> SumA21/1
  Input/1 -> s(1)/1

== stateflow chart Get_Horizontal_Measures/Measures for Offset_Calculation/CheckSum Pre-Processing/Accelerometer Processing/CheckSum Correction/Generate Sample Holding Pulse/Chart ==
  state Begin_State0
    entry: output =0;
  state Begin_State
    entry: output =1;
  state End_State
    entry: output=0;
  (default) -> Begin_State0
  Begin_State0 -> Begin_State : [if_transition==1]
  Begin_State -> End_State [order 1] : after(HoldDataTicks,tick)
  End_State -> Begin_State : [if_transition==1]
  Begin_State -> Begin_State [order 2] : [if_transition==1]
  data: output output; if_transition input; HoldDataTicks input

== stateflow chart Get_Horizontal_Measures/Measures for Offset_Calculation/CheckSum Pre-Processing/RateGyro Processing/CheckSum Correction/Generate Sample Holding Pulse/Chart ==
  state Begin_State0
    entry: output =0;
  state Begin_State
    entry: output =1;
  state End_State
    entry: output=0;
  (default) -> Begin_State0
  Begin_State0 -> Begin_State : [if_transition==1]
  Begin_State -> End_State [order 1] : after(HoldDataTicks,tick)
  End_State -> Begin_State : [if_transition==1]
  Begin_State -> Begin_State [order 2] : [if_transition==1]
  data: output output; if_transition input; HoldDataTicks input

== stateflow chart Get_Horizontal_Measures/Measures for Offset_Calculation/CheckSum Pre-Processing/Magnetometer/CheckSum Correction/Generate Sample Holding Pulse/Chart ==
  state Begin_State0
    entry: output =0;
  state Begin_State
    entry: output =1;
  state End_State
    entry: output=0;
  (default) -> Begin_State0
  Begin_State0 -> Begin_State : [if_transition==1]
  Begin_State -> End_State [order 1] : after(HoldDataTicks,tick)
  End_State -> Begin_State : [if_transition==1]
  Begin_State -> Begin_State [order 2] : [if_transition==1]
  data: output output; if_transition input; HoldDataTicks input

== stateflow chart Get_Horizontal_Measures/Measures for Offset_Calculation/CheckSum Pre-Processing/Ultrasound Processing/CheckSum Correction/Generate Sample Holding Pulse/Chart ==
  state Begin_State0
    entry: output =0;
  state Begin_State
    entry: output =1;
  state End_State
    entry: output=0;
  (default) -> Begin_State0
  Begin_State0 -> Begin_State : [if_transition==1]
  Begin_State -> End_State [order 1] : after(HoldDataTicks,tick)
  End_State -> Begin_State : [if_transition==1]
  Begin_State -> Begin_State [order 2] : [if_transition==1]
  data: output output; if_transition input; HoldDataTicks input

== stateflow chart Get_Horizontal_Measures/Measures for Offset_Calculation/CheckSum Pre-Processing/TempFilter/CheckSum Correction/Generate Sample Holding Pulse/Chart ==
  state Begin_State0
    entry: output =0;
  state Begin_State
    entry: output =1;
  state End_State
    entry: output=0;
  (default) -> Begin_State0
  Begin_State0 -> Begin_State : [if_transition==1]
  Begin_State -> End_State [order 1] : after(HoldDataTicks,tick)
  End_State -> Begin_State : [if_transition==1]
  Begin_State -> Begin_State [order 2] : [if_transition==1]
  data: output output; if_transition input; HoldDataTicks input

== matlab function Get_Horizontal_Measures/Measures for Offset_Calculation/CheckSum Pre-Processing/Ultrasound Processing/Height Calculation ==
  data: u input double; y output double; prev_good_height output double; z_1 input double
function [y,prev_good_height] = fcn(u,z_1)
%#codegen



if u<10000
    
    height = ((u - 880) /26.553);
    prev_good_height = height;
else
    
%     height = u;
%     prev_good_height = height;
    height =  z_1;
    prev_good_height = z_1; 
end

y = height;

== stateflow chart Get_Horizontal_Measures/Offset Calculation ==
  state WaitForHost [parallel]
    entry:
    reset_offset_calc = 0;
    settings: executionOrder=1
    note: Description:
        | -This state will wait for the host command to take off, while initializing the offsets (accel & gyro)
        |
        | -Upon entry, this block will set the motor to NOT ARMED (turn off integrators in controller, set safety clamp of motors to OFF)
        | -Upon entry, set the refHeight to ZERO
        | -Upon entry, reset the offset calculation such that we can re-start the averaging block
    state converge = checkConvergence(Euler_Angles) [function]
    state move = checkMove(Euler_Angles) [function]
    state Attitude_Convergence_Wait
      entry:
      initDone=false;
      during:
      Converge_Flag = checkConvergence(Gyro_Measures_for_Offset);
    state Calculate_Attitude_Offset
      entry:
      reset_offset_calc = 0 ;
      Move = false;
      during:
      Offset_Accel_Current =Accel_Offset_Calculation(Accel_Measures_for_Offset,reset_offset_calc);
      Offset_Gyro_Current =Gyro_Offset_Calculation(Gyro_Measures_for_Offset,reset_offset_calc);
      Move = checkMove(Gyro_Measures_for_Offset);
    state Auto_Calibration_Done
      entry:
      Accelerometer_Offset_Values = Offset_Accel_Current;
      Gyrometer_Offset_Values = Offset_Gyro_Current;
      reset_offset_calc = 1;
      Accel_Offset_Calculation(Accel_Measures_for_Offset,reset_offset_calc);
      Gyro_Offset_Calculation(Gyro_Measures_for_Offset,reset_offset_calc);
      during:
      initDone = true;
    (default) -> Attitude_Convergence_Wait
    Calculate_Attitude_Offset -> Attitude_Convergence_Wait [order 2] : [Move == 1 && after(0.1,sec)]
        | {reset_offset_calc = 1;
        | Accel_Offset_Calculation(Accel_Measures_for_Offset,reset_offset_calc);
        | Gyro_Offset_Calculation(Gyro_Measures_for_Offset,reset_offset_calc)}
    Attitude_Convergence_Wait -> Calculate_Attitude_Offset : [Converge_Flag==1 && after(0.1,sec)]
    Calculate_Attitude_Offset -> Auto_Calibration_Done [order 1] : [Move == 0 && after(3,sec)]
    Auto_Calibration_Done -> Calculate_Attitude_Offset : [initDone == 1 && after(0.1,sec)]
  data: Euler_Angles function_input double size=3; converge function_output; OffsetMeasure function_input; Reset function_input; Y function_output; OffsetMeasure function_input; Reset function_input; Y function_output; Euler_Angles function_input double size=3; move function_output; initDone local; Converge_Flag local; reset_offset_calc local; Accel_Measures_for_Offset input size=3; Gyro_Measures_for_Offset input size=3; Offset_Gyro_Current local; Offset_Value_Current local; Offset_Accel_Current local double; Move local; Accelerometer_Offset_Values output; Gyrometer_Offset_Values output
  data initDone settings: description=A flag to check whether the calibration is done.
  function Y = Accel_Offset_Calculation(OffsetMeasure,Reset):
    | function Y = Accel_Offset_Calculation(OffsetMeasure,Reset)
    |  
    | %Compute running average while in this state. Assumed inputs
    | %are accelerometer offset values. These values are accumulated over time
    | %and divided by the total time increment to return an average values
    | Y = [0 0 0]';
    | persistent A_x_sum
    | persistent A_y_sum
    | persistent A_z_sum
    | persistent Tick
    | 
    | if(isempty(A_x_sum) || Reset==1)
    |     A_x_sum = 0;
    |     A_y_sum = 0;
    |     A_z_sum = 0;
    |     Tick = 1;
    |         
    | else
    |     
    |     Measure_X = OffsetMeasure(1);
    |     Measure_Y = OffsetMeasure(2);
    |     Measure_Z = OffsetMeasure(3);
    | 
    |     A_x_sum = A_x_sum + Measure_X;
    |     A_y_sum = A_y_sum + Measure_Y;
    |     A_z_sum = A_z_sum + Measure_Z;
    | 
    | 
    |     Y = [A_x_sum A_y_sum A_z_sum]'./Tick;
    | 
    | 
    |     Tick = Tick + 1;
    | 
    | end
    | 
    | 
    | 
    | 
    | end
  function Y = Gyro_Offset_Calculation(OffsetMeasure,Reset):
    | function Y = Gyro_Offset_Calculation(OffsetMeasure,Reset)
    |  
    | %Compute running average while in this state. Assumed inputs
    | %are gyro offset values when drone is perfectly stationary on the ground. These values are accumulated over time
    | %and divided by the total time increment to return an average values
    | Y = [0 0 0]';
    | persistent G_x_sum
    | persistent G_y_sum
    | persistent G_z_sum
    | persistent Tick
    | 
    | if(isempty(G_x_sum) || Reset==1)
    |     G_x_sum = 0;
    |     G_y_sum = 0;
    |     G_z_sum = 0;
    | 
    |     Tick = 1;
    |         
    | else
    |     
    |     Measure_X = OffsetMeasure(1);
    |     Measure_Y = OffsetMeasure(2);
    |     Measure_Z = OffsetMeasure(3);
    | 
    |     G_x_sum = G_x_sum + Measure_X;
    |     G_y_sum = G_y_sum + Measure_Y;
    |     G_z_sum = G_z_sum + Measure_Z;
    | 
    | 
    |     Y = [G_x_sum G_y_sum G_z_sum]'./Tick;
    | 
    | 
    |     Tick = Tick + 1;
    | 
    | end
    | 
    | 
    | 
    | 
    | end
